simulink model "biciclo_FL"  (R2020a)
settings: Solver=FixedStepAuto  StartTime=0.0  StopTime=Inf  FixedStep=0.001  MaxStep=0.01  RelTol=1e-3
InitFcn:
  | init_biciclo
StopFcn:
  | stop_biciclo
values from neighbouring files (symbols this model uses):
  K1 = [20; 20]    [init_biciclo.m]
  K2 = [100; 100]    [init_biciclo.m]
  K3 = [10; 10]    [init_biciclo.m]
  L = 1    [init_biciclo.m]
  Lsofar = [Lsofar; sum(Lenghts)]    [init_biciclo.m]
  Ltot = sum(Lenghts)    [init_biciclo.m]
  n_p = length(points)    [init_biciclo.m]
  phi_iniziale = pi/18    (= 0.174532925199)    [init_biciclo.m]
  theta_P_iniziale = 0    [init_biciclo.m]
  theta_rette = [theta_rette ; theta_rette(n_p-2)+pi]    [init_biciclo.m]
  v_P_dot_iniziale = 0.1    [init_biciclo.m]
  v_P_iniziale = 1    [init_biciclo.m]
  x_M_finale = points(1)    [init_biciclo.m]
  x_M_iniziale = x_M_iniziale + offset_iniziale    (= 0.5)    [init_biciclo.m]
  xp = points(:,1)    [init_biciclo.m]
  y_M_finale = points(2)    [init_biciclo.m]
  y_M_iniziale = y_M_iniziale + offset_iniziale*2    (= 1)    [init_biciclo.m]
  yp = points(:,2)    [init_biciclo.m]
undefined symbols (not defined in the file or in its folder): indexclot, Lsofarclot
libraries: simulink x1
settings Model: Creator=Andrea_Ferroni  LastModifiedBy=Francesco

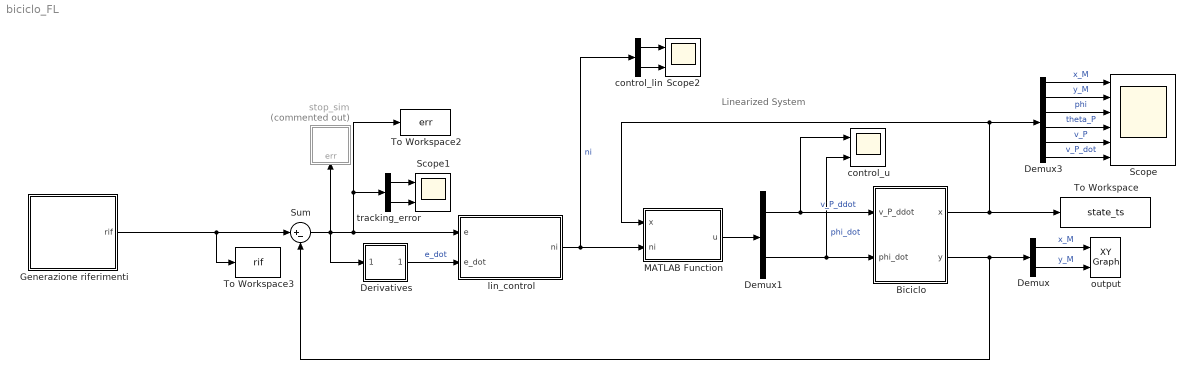
== system biciclo_FL ==
  note: Linearized System
  Biciclo : Subsystem
  Demux : Demux  Outputs=2
  Demux1 : Demux  Outputs=2
  Demux3 : Demux  Outputs=6
  Derivatives : Subsystem
  Generazione riferimenti : Subsystem  Variant=on
  MATLAB Function : MATLAB Function  TreatAsAtomicUnit=on
  Scope : Scope  NumInputPorts=6
  Scope1 : Scope  NumInputPorts=2
  Scope2 : Scope  NumInputPorts=2
  Sum : Sum  Inputs=|+-
  To Workspace : ToWorkspace  VariableName=state_ts  SaveFormat=Timeseries  SampleTime=-1
  To Workspace2 : ToWorkspace  VariableName=err  SaveFormat=Timeseries  SampleTime=-1
  To Workspace3 : ToWorkspace  VariableName=rif  SaveFormat=Timeseries  SampleTime=-1
  control_lin : Demux  Outputs=2
  control_u : Scope  NumInputPorts=2
  lin_control : MATLAB Function  TreatAsAtomicUnit=on
  output : simulink/Sinks/XY Graph  xmin=-50  xmax=50  ymin=-50  ymax=50  st=-1
  stop_sim : Subsystem  Commented=on
  tracking_error : Demux  Outputs=2
  wires:
  Biciclo/1(x) -> To Workspace/1, Demux3/1, MATLAB Function/1(x)
  Biciclo/2(y) -> Demux/1, Sum/2
  lin_control/1(ni) -> control_lin/1, MATLAB Function/2(ni)  "ni"
  Sum/1 -> Derivatives/1(In1), lin_control/1(e), tracking_error/1, To Workspace2/1, stop_sim/1(err)
  Derivatives/1(Out1) -> lin_control/2(e_dot)  "e_dot"
  Demux/1 -> output/1  "x_M"
  Demux/2 -> output/2  "y_M"
  tracking_error/1 -> Scope1/1
  tracking_error/2 -> Scope1/2
  MATLAB Function/1(u) -> Demux1/1
  Demux1/1 -> control_u/1, Biciclo/1(v_P_ddot)  "v_P_ddot"
  Demux1/2 -> control_u/2, Biciclo/2(phi_dot)  "phi_dot"
  control_lin/2 -> Scope2/2
  control_lin/1 -> Scope2/1
  Demux3/1 -> Scope/1  "x_M"
  Demux3/2 -> Scope/2  "y_M"
  Demux3/3 -> Scope/3  "phi"
  Demux3/4 -> Scope/4  "theta_P"
  Demux3/6 -> Scope/6  "v_P_dot"
  Demux3/5 -> Scope/5  "v_P"
  Generazione riferimenti/1(rif) -> To Workspace3/1, Sum/1

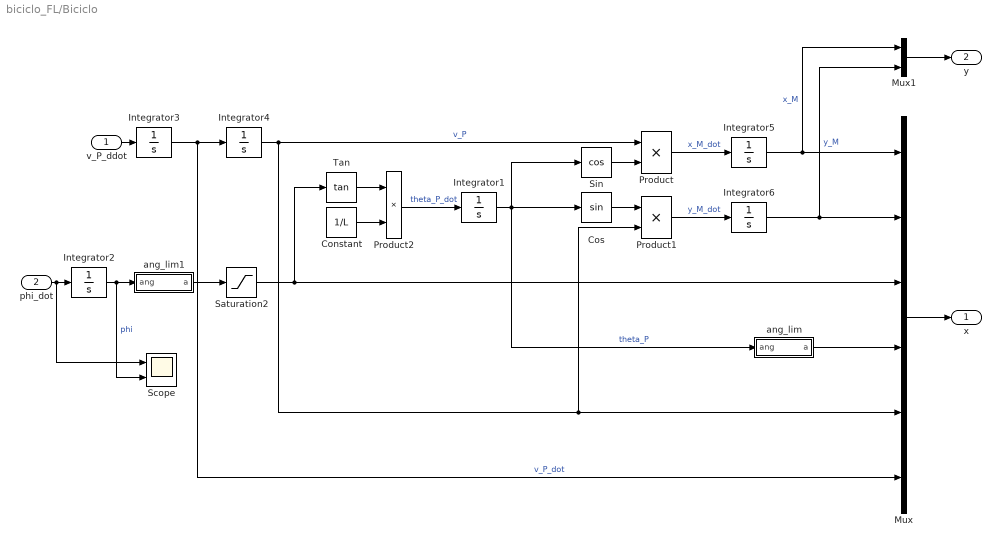
== system biciclo_FL/Biciclo ==
  v_P_ddot : Inport
  phi_dot : Inport  Port=2
  Constant : Constant  Value=1/L
  Cos : Trigonometry
  Integrator1 : Integrator  InitialCondition=theta_P_iniziale
  Integrator2 : Integrator  InitialCondition=phi_iniziale  LimitOutput=on  UpperSaturationLimit=pi/2  LowerSaturationLimit=-pi/2
  Integrator3 : Integrator  InitialCondition=v_P_dot_iniziale
  Integrator4 : Integrator  InitialCondition=v_P_iniziale
  Integrator5 : Integrator  InitialCondition=x_M_iniziale
  Integrator6 : Integrator  InitialCondition=y_M_iniziale
  Mux : Mux  Inputs=6
  Mux1 : Mux  Inputs=2
  Product : Product
  Product1 : Product
  Product2 : Product
  Saturation2 : Saturate  UpperLimit=pi/2*0.999  LowerLimit=-pi/2*0.999
  Scope : Scope  NumInputPorts=2
  Sin : Trigonometry  Operator=cos
  Tan : Trigonometry  Operator=tan
  ang_lim : MATLAB Function  TreatAsAtomicUnit=on
  ang_lim1 : MATLAB Function  TreatAsAtomicUnit=on
  x : Outport
  y : Outport  Port=2
  wires:
  v_P_ddot/1 -> Integrator3/1
  phi_dot/1 -> Scope/1, Integrator2/1
  Mux/1 -> x/1
  Integrator3/1 -> Integrator4/1, Mux/6  "v_P_dot"
  Integrator1/1 -> Sin/1, ang_lim/1(ang), Cos/1  "theta_P"
  Integrator4/1 -> Product1/2, Mux/5, Product/1  "v_P"
  Integrator2/1 -> Scope/2, ang_lim1/1(ang)  "phi"
  Sin/1 -> Product/2
  Cos/1 -> Product1/1
  Product/1 -> Integrator5/1  "x_M_dot"
  Product1/1 -> Integrator6/1  "y_M_dot"
  Tan/1 -> Product2/1
  Constant/1 -> Product2/2
  Product2/1 -> Integrator1/1  "theta_P_dot"
  Mux1/1 -> y/1
  Integrator5/1 -> Mux1/1, Mux/1  "x_M"
  Integrator6/1 -> Mux1/2, Mux/2  "y_M"
  ang_lim/1(a) -> Mux/4
  Saturation2/1 -> Mux/3, Tan/1
  ang_lim1/1(a) -> Saturation2/1

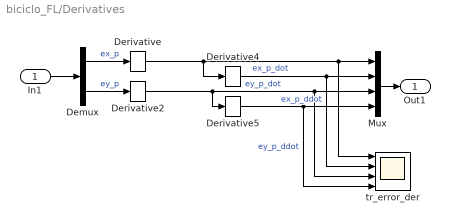
== system biciclo_FL/Derivatives ==
  In1 : Inport
  Demux : Demux  Outputs=2
  Derivative{,2,4..5} (4 alike) : Derivative  CoefficientInTFapproximation=1e10
  Mux : Mux
  tr_error_der : Scope  NumInputPorts=4
  Out1 : Outport
  wires:
  In1/1 -> Demux/1
  Demux/1 -> Derivative/1  "ex_p"
  Derivative/1 -> Derivative4/1, tr_error_der/1, Mux/1  "ex_p_dot"
  Demux/2 -> Derivative2/1  "ey_p"
  Mux/1 -> Out1/1
  Derivative4/1 -> tr_error_der/2, Mux/2  "ex_p_ddot"
  Derivative2/1 -> Derivative5/1, tr_error_der/3, Mux/3  "ey_p_dot"
  Derivative5/1 -> tr_error_der/4, Mux/4  "ey_p_ddot"

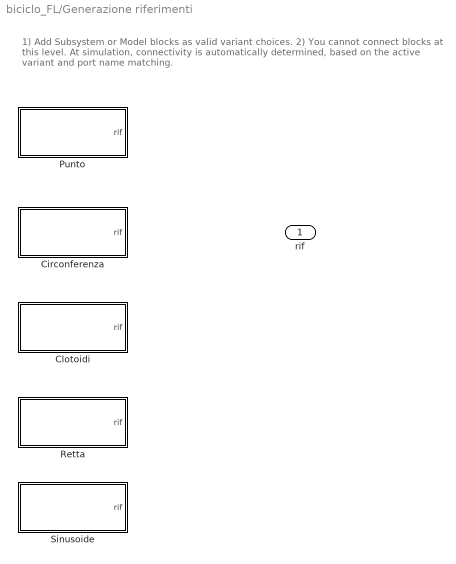
== system biciclo_FL/Generazione riferimenti ==
  note: 1) Add Subsystem or Model blocks as valid variant choices.
      | 2) You cannot connect blocks at this level. At simulation, connectivity is automatically
      | determined, based on the active variant and port name matching.
  Circonferenza : Subsystem  VariantControl=Circonferenza
  Clotoidi : Subsystem  VariantControl=Clotoidi
  Punto : Subsystem  VariantControl=Punto
  Retta : Subsystem  VariantControl=Retta
  Sinusoide : Subsystem  VariantControl=Sinusoide
  rif : Outport

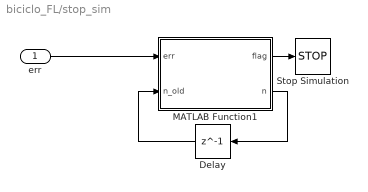
== system biciclo_FL/stop_sim ==
  err : Inport
  Delay : Delay  DelayLength=1
  MATLAB Function1 : MATLAB Function  TreatAsAtomicUnit=on
  Stop Simulation : Stop
  wires:
  MATLAB Function1/2(n) -> Delay/1
  MATLAB Function1/1(flag) -> Stop Simulation/1
  err/1 -> MATLAB Function1/1(err)
  Delay/1 -> MATLAB Function1/2(n_old)

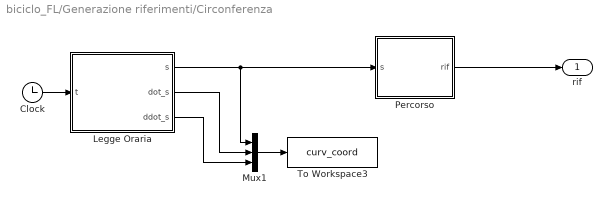
== system biciclo_FL/Generazione riferimenti/Circonferenza ==
  Clock : Clock
  Legge Oraria : MATLAB Function  TreatAsAtomicUnit=on
  Mux1 : Mux  Inputs=3
  Percorso : MATLAB Function  TreatAsAtomicUnit=on
  To Workspace3 : ToWorkspace  VariableName=curv_coord  SaveFormat=Timeseries  SampleTime=-1
  rif : Outport
  wires:
  Legge Oraria/2(dot_s) -> Mux1/2
  Clock/1 -> Legge Oraria/1(t)
  Mux1/1 -> To Workspace3/1
  Legge Oraria/3(ddot_s) -> Mux1/3
  Legge Oraria/1(s) -> Percorso/1(s), Mux1/1
  Percorso/1(rif) -> rif/1

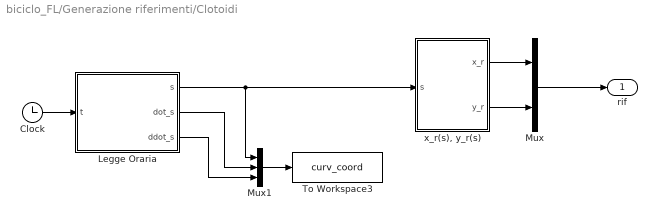
== system biciclo_FL/Generazione riferimenti/Clotoidi ==
  Clock : Clock
  Legge Oraria : MATLAB Function  TreatAsAtomicUnit=on
  Mux : Mux  Inputs=2
  Mux1 : Mux  Inputs=3
  To Workspace3 : ToWorkspace  VariableName=curv_coord  SaveFormat=Timeseries  SampleTime=-1
  "x_r(s), y_r(s)" : MATLAB Function  TreatAsAtomicUnit=on
  rif : Outport
  wires:
  Legge Oraria/1(s) -> Mux1/1, "x_r(s), y_r(s)"/1(s)
  Legge Oraria/2(dot_s) -> Mux1/2
  Clock/1 -> Legge Oraria/1(t)
  Legge Oraria/3(ddot_s) -> Mux1/3
  Mux1/1 -> To Workspace3/1
  "x_r(s), y_r(s)"/2(y_r) -> Mux/2
  "x_r(s), y_r(s)"/1(x_r) -> Mux/1
  Mux/1 -> rif/1

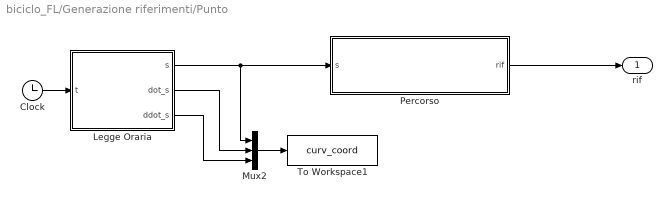
== system biciclo_FL/Generazione riferimenti/Punto ==
  Clock : Clock
  Legge Oraria : MATLAB Function  TreatAsAtomicUnit=on
  Mux2 : Mux  Inputs=3
  Percorso : MATLAB Function  TreatAsAtomicUnit=on
  To Workspace1 : ToWorkspace  VariableName=curv_coord  SaveFormat=Timeseries  SampleTime=-1
  rif : Outport
  wires:
  Legge Oraria/2(dot_s) -> Mux2/2
  Clock/1 -> Legge Oraria/1(t)
  Mux2/1 -> To Workspace1/1
  Legge Oraria/3(ddot_s) -> Mux2/3
  Legge Oraria/1(s) -> Mux2/1, Percorso/1(s)
  Percorso/1(rif) -> rif/1

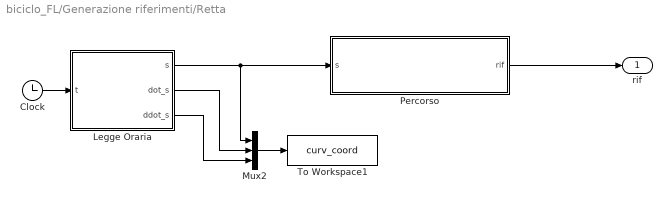
== system biciclo_FL/Generazione riferimenti/Retta ==
  Clock : Clock
  Legge Oraria : MATLAB Function  TreatAsAtomicUnit=on
  Mux2 : Mux  Inputs=3
  Percorso : MATLAB Function  TreatAsAtomicUnit=on
  To Workspace1 : ToWorkspace  VariableName=curv_coord  SaveFormat=Timeseries  SampleTime=-1
  rif : Outport
  wires:
  Percorso/1(rif) -> rif/1
  Legge Oraria/1(s) -> Percorso/1(s), Mux2/1
  Legge Oraria/3(ddot_s) -> Mux2/3
  Mux2/1 -> To Workspace1/1
  Clock/1 -> Legge Oraria/1(t)
  Legge Oraria/2(dot_s) -> Mux2/2

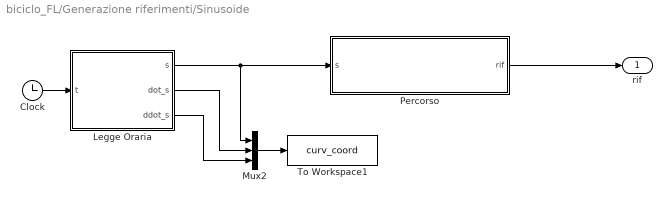
== system biciclo_FL/Generazione riferimenti/Sinusoide ==
  Clock : Clock
  Legge Oraria : MATLAB Function  TreatAsAtomicUnit=on
  Mux2 : Mux  Inputs=3
  Percorso : MATLAB Function  TreatAsAtomicUnit=on
  To Workspace1 : ToWorkspace  VariableName=curv_coord  SaveFormat=Timeseries  SampleTime=-1
  rif : Outport
  wires:
  Legge Oraria/2(dot_s) -> Mux2/2
  Clock/1 -> Legge Oraria/1(t)
  Mux2/1 -> To Workspace1/1
  Legge Oraria/3(ddot_s) -> Mux2/3
  Legge Oraria/1(s) -> Mux2/1, Percorso/1(s)
  Percorso/1(rif) -> rif/1

== matlab function biciclo_FL/Biciclo/ang_lim1 ==
  data: ang input; a output
function a = ang_lim(ang)

	c = cos(ang);
	s = sin(ang);
	a = atan2(s, c);

end

== matlab function biciclo_FL/Generazione riferimenti/Circonferenza/Legge Oraria ==
  data: t input; s output; v_rif parameter; dot_s output; ddot_s output
function [s, dot_s, ddot_s]  = legge_oraria(t, v_rif)
%#codegen PEPO

s = v_rif*t;
dot_s = v_rif;
ddot_s = 0.0;


end

== matlab function biciclo_FL/Generazione riferimenti/Circonferenza/Percorso ==
  data: s input; rif output; centro parameter
function rif = percorso(s, centro)


r = 1;
theta_circ = s/r;

if theta_circ >=  3*2*pi % dopotre giri ti fermi
	theta_circ = 3*2*pi;
end

rif = centro + r*[cos(theta_circ);sin(theta_circ)];		% circonferenza

end

== matlab function biciclo_FL/Generazione riferimenti/Retta/Legge Oraria ==
  data: t input; s output; v_rif parameter; dot_s output; ddot_s output
function [s, dot_s, ddot_s]  = legge_oraria(t, v_rif)
%#codegen PEPO

s = v_rif*t;
dot_s = v_rif;
ddot_s = 0.0;


end

== matlab function biciclo_FL/Generazione riferimenti/Retta/Percorso ==
  data: s input; rif output; dir_retta parameter
function rif  = retta(s, dir_retta)

rif = [0;0] + s * dir_retta;


end

== matlab function biciclo_FL/Generazione riferimenti/Clotoidi/x_r(s), y_r(s) ==
  data: s input; x_r output size=1; y_r output size=1; indexclot parameter; theta_rette parameter; yp parameter; xp parameter; Lsofar parameter; n_p parameter; Lsofarclot parameter; Ltot parameter
function [x_r,y_r] = percorso(s, indexclot, theta_rette, yp, xp, ...
										Lsofar, n_p, Lsofarclot, Ltot)
									
coder.extrinsic('pointsOnClothoid')
% fine percorso
if s >= Ltot
	s = Ltot; % cosi` da plottare l'ultimo punto
end

ntratto=0;
	XYS = [0; 0]; %definito prima

	%Parte per capire in che tratto sono
	if s < Lsofar(1)
		ntratto=1;
	else
		for ii=2:(n_p-1)
			if s>=Lsofar(ii-1) && s<=Lsofar(ii)
				ntratto=ii;
			end
		end
	end	

		%calcolo delle coordinate x e y riferite a s e a ntratto
	if mod(ntratto,2)==1            %tratti dispari - rette
		if ntratto==1
			XYS=[xp(ntratto)+cos(theta_rette(ntratto))*(s); ...
				yp(ntratto)+sin(theta_rette(ntratto))*(s)];
		else
			srel=s-Lsofar(ntratto-1);
			XYS=[	xp(ntratto)	+ cos(theta_rette(ntratto))	* srel; ...
					yp(ntratto)	+ sin(theta_rette(ntratto))	* srel];
		end 

	elseif mod(ntratto,2)==0	%tratti pari - clotoidi
		srel=s-Lsofar(ntratto-1);

		if srel<=Lsofarclot(ntratto/2).Lclot(1)
			XYS = double(pointsOnClothoid( indexclot(ntratto/2).clot.S0, srel ));

		elseif srel>Lsofarclot(ntratto/2).Lclot(1) & srel<=Lsofarclot(ntratto/2).Lclot(2)
			XYS = double(pointsOnClothoid( indexclot(ntratto/2).clot.SM, srel- indexclot(ntratto/2).clot.S0.L ));

		elseif srel>Lsofarclot(ntratto/2).Lclot(2)
			XYS = double(pointsOnClothoid( indexclot(ntratto/2).clot.S1, srel- indexclot(ntratto/2).clot.S0.L - indexclot(ntratto/2).clot.SM.L ));
		end

		%XYS = double(pointsOnClothoid( indexclot(ntratto/2).clot, s-Lsofar(ntratto-1) ));
	end

	x_r = XYS(1);
	y_r = XYS(2);
%--------------------------------------------------
% end function
end

== matlab function biciclo_FL/Generazione riferimenti/Sinusoide/Legge Oraria ==
  data: t input; s output; v_rif parameter; dot_s output; ddot_s output
function [s, dot_s, ddot_s]  = legge_oraria(t, v_rif)
%#codegen PEPO

s = v_rif*t;
dot_s = v_rif;
ddot_s = 0.0;


end

== matlab function biciclo_FL/Generazione riferimenti/Sinusoide/Percorso ==
  data: s input; rif output; dir_retta parameter
function rif  = retta(s, dir_retta)

r = 5;
theta_circ = s/r;

% if theta_circ >=  3*2*pi % dopotre giri ti fermi
% 	theta_circ = 3*2*pi;
% end

rif = dir_retta * s + r*[0; sin(theta_circ)];	% circonferenza

end

== matlab function biciclo_FL/lin_control ==
  data: e input; ni output; e_dot input; K1 parameter; K2 parameter; K3 parameter
function ni = lin_control(e, e_dot, K1, K2, K3)


edot = e_dot([1,3],1);
eddot = e_dot([2,4],1);

ni = K1.*e + K2.*edot + K3.*eddot;


end

== matlab function biciclo_FL/MATLAB Function ==
  data: x input; ni input; u output; L parameter
function u = Linearized(x,ni,L)
E_inv = inv_E(x,L);
G = Gamma(x,L);
u =  -E_inv*G + E_inv*ni;
end

% gamma
function Gm = Gamma(x,L)
phi = x(3);
theta_P = x(4);
v_P = x(5);
v_P_dot = x(6);

Gm =  [- (v_P*tan(phi)*((cos(theta_P)*tan(phi)*v_P^2)/L + v_P_dot*sin(theta_P)))/L - (2*v_P*v_P_dot*tan(phi)*sin(theta_P))/L;...
		 (v_P*tan(phi)*(v_P_dot*cos(theta_P) - (v_P^2*tan(phi)*sin(theta_P))/L))/L + (2*v_P*v_P_dot*cos(theta_P)*tan(phi))/L];
end
% 
function E_in = inv_E(x,L)
phi = x(3);
theta_P = x(4);
v_P = x(5);

E =[cos(theta_P), -(v_P^2*sin(theta_P)*(tan(phi)^2 + 1))/L;	sin(theta_P),  (v_P^2*cos(theta_P)*(tan(phi)^2 + 1))/L];


% if rcond(E) < 1e-5
% 	ciao = 1;
% end

E_in = inv(E);


end

== matlab function biciclo_FL/Generazione riferimenti/Punto/Legge Oraria ==
  data: t input; s output; v_rif parameter; dot_s output; ddot_s output
function [s, dot_s, ddot_s]  = legge_oraria(t, v_rif)
%#codegen PEPO

s = v_rif*t;
dot_s = v_rif;
ddot_s = 0.0;


end

== matlab function biciclo_FL/Biciclo/ang_lim ==
  data: ang input; a output
function a = ang_lim(ang)

	c = cos(ang);
	s = sin(ang);
	a = atan2(s, c);

end

== matlab function biciclo_FL/stop_sim/MATLAB Function1 ==
  data: flag output; err input; n output; n_old input; threshold parameter
function [flag, n] = stop_function(err, n_old, threshold)
	flag = 0;
	n = n_old;
	if norm(err, 2) < threshold
		n=n+1;
	else
		n=0;
	end
	
	if n > 500
		flag = 1;
		n = 0;
	end
end

== matlab function biciclo_FL/Generazione riferimenti/Punto/Percorso ==
  data: s input; rif output; x_M_finale parameter; x_M_iniziale parameter; y_M_finale parameter; y_M_iniziale parameter
function rif  = punto2punto(s, x_M_finale, x_M_iniziale, y_M_finale, y_M_iniziale)

vett = [x_M_finale - x_M_iniziale; y_M_finale - y_M_iniziale];
Ltot = norm(vett,2);
direzione = vett/Ltot;
offset = 0;

if s >= Ltot
	rif = [x_M_finale + offset; y_M_finale + offset];
else
	rif = [ x_M_iniziale + offset; y_M_iniziale + offset] + s * direzione;
end
% 
% if s > 2*Ltot
% 	s = mod(s, 2*Ltot);
% end
% 
% if s >= Ltot
% 	rif = [ x_M_finale ; y_M_finale ] - (s-Ltot) * direzione;
% 	
% else
% 	rif = [ x_M_iniziale ; y_M_iniziale ] + s * direzione;
% end



end

== matlab function biciclo_FL/Generazione riferimenti/Clotoidi/Legge Oraria ==
  data: t input; s output; v_rif parameter; dot_s output; ddot_s output
function [s, dot_s, ddot_s]  = legge_oraria(t, v_rif)
%#codegen PEPO

s = v_rif*t;
dot_s = v_rif;
ddot_s = 0.0;


end
